simulink model "RRR_l5controller2"  (R2020a)
settings: Solver=ode3  StartTime=0.0  StopTime=2.1  RelTol=1e-3
libraries: roblocks x4
settings Model: Creator=yrza  LastModifiedBy=angelina

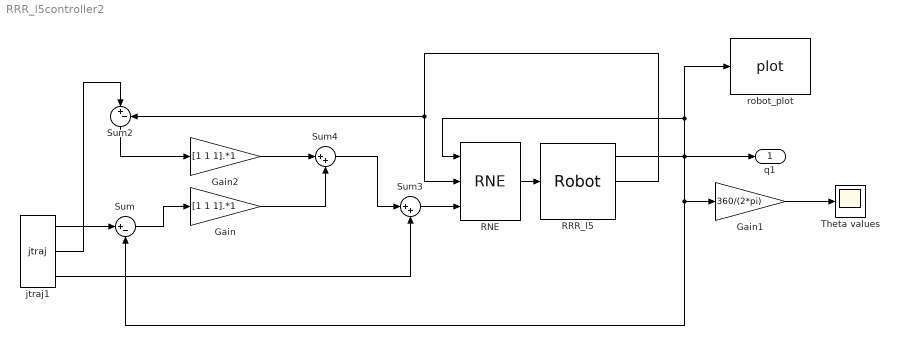
== system RRR_l5controller2 ==
  Gain : Gain  Gain=[1 1 1].*1
  Gain1 : Gain  Gain=360/(2*pi)
  Gain2 : Gain  Gain=[1 1 1].*1
  RNE : roblocks/Arm/RNE  robot=RRR_l5  grav=[0 0 9.81]
  RRR_l5 : roblocks/Arm/Robot  robot=RRR_l5  q0=[0 0 0]
  Sum : Sum  Inputs=|+-
  Sum2 : Sum  Inputs=|+-
  Sum3 : Sum  Inputs=|++
  Sum4 : Sum  Inputs=|++
  Theta values : Scope
  jtraj1 : roblocks/Toolbox/jtraj  q0=[0 0 0]  qf=[pi/2 -pi/4 -pi/4]  tmax=2  ts=0.02
  robot_plot : roblocks/Arm/plot  robot=RRR_l5  fps=10  holdplot=on
  q1 : Outport
  wires:
  RRR_l5/1 -> q1/1, robot_plot/1, RNE/1, Gain1/1, Sum/2
  Gain1/1 -> Theta values/1
  jtraj1/1 -> Sum/1
  RRR_l5/2 -> RNE/2, Sum2/2
  Gain/1 -> Sum4/2
  Sum/1 -> Gain/1
  RNE/1 -> RRR_l5/1
  jtraj1/2 -> Sum2/1
  jtraj1/3 -> Sum3/2
  Sum4/1 -> Sum3/1
  Sum3/1 -> RNE/3
  Sum2/1 -> Gain2/1
  Gain2/1 -> Sum4/1
